simulink model "MRAC_111"  (Simulink 8.5)
settings: Solver=ode45  SolverMode=SingleTasking  StartTime=10  StopTime=20  RelTol=1e-3  AbsTol=1e-6
values from neighbouring files (symbols this model uses):
  As = 0    [parameters.m]    (also in simu01.m; simu02.m; simu03.m; simu04.m)
  DC = 1    [parameters.m]    (also in simu01.m; simu02.m; simu03.m; simu04.m)
  gamma = 10    [parameters.m]    (also in simu01.m = 100; simu02.m = 100; simu03.m = 100; simu04.m)
  st = 0.05    [parameters.m]    (also in simu01.m; simu02.m = 0.01; simu03.m = 0.001; simu04.m)
  theta0 = 0    [parameters.m]    (also in simu01.m; simu02.m; simu03.m; simu04.m)
  ws = 10    [parameters.m]    (also in simu01.m; simu02.m; simu03.m = 1; simu04.m)
libraries: cstblocks x2
settings Model: Creator=Ramon  LastModifiedBy=ramon
settings DataIOCC: LimitDataPoints=off  SaveOutput=off  SaveTime=off
settings OptimizationCC: BlockReduction=off  BooleanDataType=off  InitFltsAndDblsToZero=on
settings DebuggingCC: SaveWithParameterizedLinksMsg=none  SignalResolutionControl=TryResolveAllWithWarning  MultiTaskDSMMsg=warning  MultiTaskCondExecSysMsg=none  FcnCallInpInsideContextMsg=UseLocalSettings
settings HardwareCC: TargetUnknown=on
settings RTWCC: TemplateMakefile=grt_vc.tmf

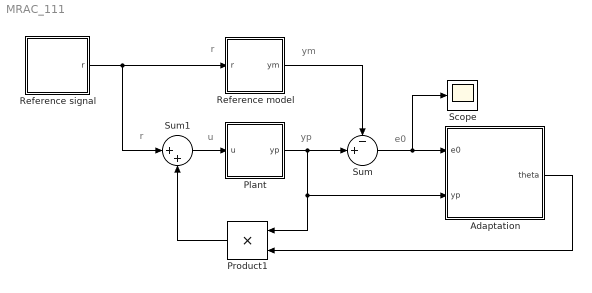
== system MRAC_111 ==
  note: u
  note: r
  note: e0
  note: yp
  note: ym
  note: r
  Adaptation : Subsystem
  Plant : Subsystem
  Product1 : Product  SaturateOnIntegerOverflow=on  RndMeth=Zero  InputSameDT=on  OutDataTypeStr=Inherit: Same as first input
  Reference model : Subsystem
  Reference signal : Subsystem
  Scope : Scope
      settings: TickLabels=on  TimeRange=20  YMin=-1  YMax=2
  Sum : Sum  Inputs=-+|  SaturateOnIntegerOverflow=on  InputSameDT=on  OutDataTypeStr=Inherit: Same as first input
  Sum1 : Sum  Inputs=|++  SaturateOnIntegerOverflow=on  InputSameDT=on  OutDataTypeStr=Inherit: Same as first input
  wires:
  Sum/1 -> Adaptation/1(e0), Scope/1
  Reference model/1(ym) -> Sum/1
  Plant/1(yp) -> Sum/2, Adaptation/2(yp), Product1/1
  Reference signal/1(r) -> Reference model/1(r), Sum1/1
  Sum1/1 -> Plant/1(u)
  Adaptation/1(theta) -> Product1/2
  Product1/1 -> Sum1/2

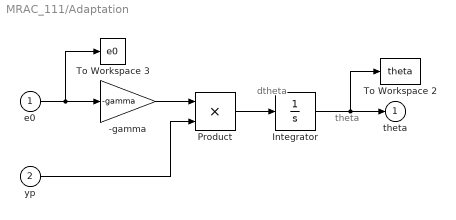
== system MRAC_111/Adaptation ==
  note: theta
  note: dtheta
  e0 : Inport  PortDimensions=1
  yp : Inport  Port=2
  -gamma : Gain  Gain=-gamma  SaturateOnIntegerOverflow=on  OutDataTypeStr=Inherit: Same as input  ParamDataTypeStr=Inherit: Same as input
  Integrator : Integrator  InitialCondition=theta0
  Product : Product  SaturateOnIntegerOverflow=on  RndMeth=Zero  InputSameDT=on  OutDataTypeStr=Inherit: Same as first input
  To Workspace 2 : ToWorkspace  VariableName=theta  SampleTime=st
  To Workspace 3 : ToWorkspace  VariableName=e0  SampleTime=st
  theta : Outport  InitialOutput=0
  wires:
  Integrator/1 -> To Workspace 2/1, theta/1
  -gamma/1 -> Product/1
  yp/1 -> Product/2
  e0/1 -> To Workspace 3/1, -gamma/1
  Product/1 -> Integrator/1

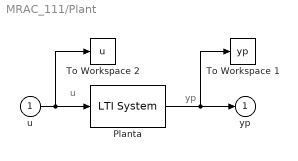
== system MRAC_111/Plant ==
  note: yp
  note: u
  u : Inport
  Planta : cstblocks/LTI System  sys=P  IC=x0
  To Workspace 1 : ToWorkspace  VariableName=yp  SampleTime=st
  To Workspace 2 : ToWorkspace  VariableName=u  SampleTime=st
  yp : Outport  InitialOutput=0
  wires:
  u/1 -> To Workspace 2/1, Planta/1
  Planta/1 -> yp/1, To Workspace 1/1

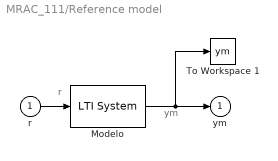
== system MRAC_111/Reference model ==
  note: r
  note: ym
  r : Inport
  Modelo : cstblocks/LTI System  sys=M  IC=xm0
  To Workspace 1 : ToWorkspace  VariableName=ym  SampleTime=st
  ym : Outport  InitialOutput=0
  wires:
  Modelo/1 -> To Workspace 1/1, ym/1
  r/1 -> Modelo/1

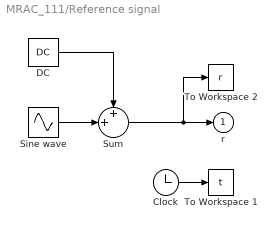
== system MRAC_111/Reference signal ==
  Clock : Clock
  DC : Constant  Value=DC
  Sine wave : Sin  Amplitude=As  Frequency=ws  SampleTime=0
  Sum : Sum  Inputs=++|  SaturateOnIntegerOverflow=on  InputSameDT=on  OutDataTypeStr=Inherit: Same as first input
  To Workspace 1 : ToWorkspace  VariableName=t  SampleTime=st
  To Workspace 2 : ToWorkspace  VariableName=r  SampleTime=st
  r : Outport  InitialOutput=0
  wires:
  DC/1 -> Sum/1
  Sum/1 -> r/1, To Workspace 2/1
  Clock/1 -> To Workspace 1/1
  Sine wave/1 -> Sum/2
